simulink model "ComponentSS"  (Simulink 7.5)
settings: Solver=ode45  StartTime=0.0  StopTime=inf  MaxStep=2e-2  RelTol=1e-3
InitFcn:
  | k1=1.5;
  | k2=.4;
  | c1=.5;
  | c2=.001;
  | m1=.1;
  | m2=.002;
  | 
  | A=[0,0,1,0;0,0,0,1;-(k1+k2)/m1,k2/m1,-(c1+c2)/m1,c2/m1;k2/m2,-k2/m2,c2/m2,-c2/m2];
  | B=[0,0;0,0;1/m1,0;0,1/m2];
  | C=eye(4);
  | D=zeros(4,2);
settings Model: Creator=cfadnavi  LastModifiedBy=dmanegol

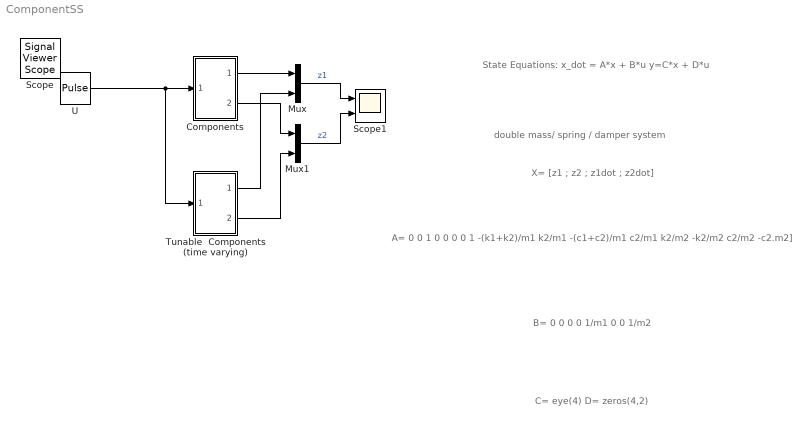
== system ComponentSS ==
  note: State Equations:
      | x_dot = A*x + B*u
      | y=C*x + D*u
  note: X=
      | [z1 ; z2 ; z1dot ; z2dot]
  note: A=
      | 0                  0                   1                 0
      | 0                  0                   0                 1
      | -(k1+k2)/m1     k2/m1   -(c1+c2)/m1    c2/m1
      | k2/m2         -k2/m2         c2/m2         -c2.m2]
  note: B=
      | 0              0
      | 0              0
      | 1/m1        0
      | 0      1/m2
  note: C= eye(4)
      |
      | D= zeros(4,2)
  note: double mass/ spring / damper system
  Components : Subsystem
  Mux : Mux  Inputs=2
  Mux1 : Mux  Inputs=2
  Scope1 : Scope  NumInputPorts=2
      settings: TimeRange=10  YMin=-0.5~-2  YMax=2.5~10
  Tunable  Components (time varying) : Subsystem
  U : DiscretePulseGenerator  PulseType=Time based  Amplitude=[1,1]  Period=[10,10]  PulseWidth=50  PhaseDelay=0  SampleTime=1
  Scope : SignalViewerScope  IOType=viewer  RefreshTime=0.035000
  wires:
  U/1 -> Components/1(In1), Tunable  Components (time varying)/1(In1)
  Components/1(Out1) -> Mux/1
  Mux/1 -> Scope1/1  "z1"
  Mux1/1 -> Scope1/2  "z2"
  Tunable  Components (time varying)/1(Out2) -> Mux/2
  Components/2(Out2) -> Mux1/1
  Tunable  Components (time varying)/2(Out3) -> Mux1/2

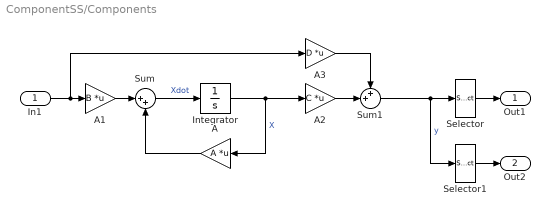
== system ComponentSS/Components ==
  In1 : Inport
  A : Gain  Gain=A  Multiplication=Matrix(K*u)  ParameterDataType=fixdt(1, 16)  ParameterScaling=2^0  OutDataType=fixdt(1, 16)  OutScaling=2^0
  A1 : Gain  Gain=B  Multiplication=Matrix(K*u)  ParameterDataType=fixdt(1, 16)  ParameterScaling=2^0  OutDataType=fixdt(1, 16)  OutScaling=2^0
  A2 : Gain  Gain=C  Multiplication=Matrix(K*u)  ParameterDataType=fixdt(1, 16)  ParameterScaling=2^0  OutDataType=fixdt(1, 16)  OutScaling=2^0
  A3 : Gain  Gain=D  Multiplication=Matrix(K*u)  ParameterDataType=fixdt(1, 16)  ParameterScaling=2^0  OutDataType=fixdt(1, 16)  OutScaling=2^0
  Integrator : Integrator
  Selector : Selector  InputPortWidth=4  IndexOptions=Index vector (dialog)  Indices=1  OutputSizes=1
  Selector1 : Selector  InputPortWidth=4  IndexOptions=Index vector (dialog)  Indices=2  OutputSizes=1
  Sum : Sum  Inputs=|++  OutDataType=fixdt(1, 16)  OutScaling=2^0
  Sum1 : Sum  Inputs=++|  OutDataType=fixdt(1, 16)  OutScaling=2^0
  Out1 : Outport
  Out2 : Outport  Port=2
  wires:
  A/1 -> Sum/2
  Integrator/1 -> A/1, A2/1  "X"
  Sum/1 -> Integrator/1  "Xdot"
  A1/1 -> Sum/1
  A2/1 -> Sum1/2
  A3/1 -> Sum1/1
  In1/1 -> A3/1, A1/1
  Sum1/1 -> Selector/1, Selector1/1  "y"
  Selector/1 -> Out1/1
  Selector1/1 -> Out2/1

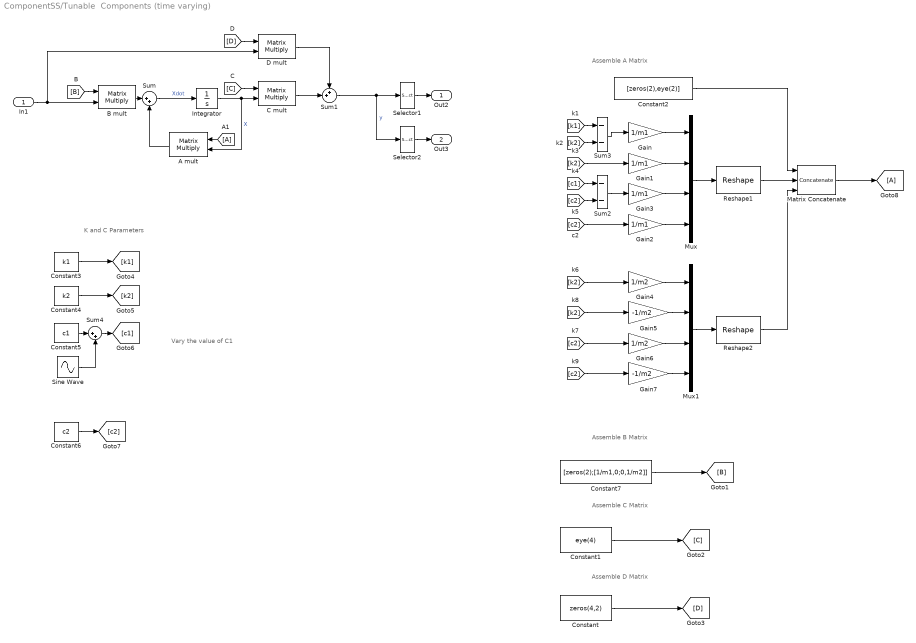
== system ComponentSS/Tunable  Components (time varying) ==
  note: Assemble A Matrix
  note: Assemble B Matrix
  note: Assemble D Matrix
  note: Assemble C Matrix
  note: K and C Parameters
  note: Vary the value of C1
  In1 : Inport
  A mult : Product  Multiplication=Matrix(*)  OutDataType=fixdt(1, 16)  OutScaling=2^0  RndMeth=Zero
  B mult : Product  Multiplication=Matrix(*)  OutDataType=fixdt(1, 16)  OutScaling=2^0  RndMeth=Zero
  C mult : Product  Multiplication=Matrix(*)  OutDataType=fixdt(1, 16)  OutScaling=2^0  RndMeth=Zero
  Constant : Constant  Value=zeros(4,2)  OutDataType=fixdt(1, 16)  OutScaling=2^0
  Constant1 : Constant  Value=eye(4)  OutDataType=fixdt(1, 16)  OutScaling=2^0
  Constant2 : Constant  Value=[zeros(2),eye(2)]  OutDataType=fixdt(1, 16)  OutScaling=2^0
  Constant3 : Constant  Value=k1  OutDataType=fixdt(1, 16)  OutScaling=2^0
  Constant4 : Constant  Value=k2  OutDataType=fixdt(1, 16)  OutScaling=2^0
  Constant5 : Constant  Value=c1  OutDataType=fixdt(1, 16)  OutScaling=2^0
  Constant6 : Constant  Value=c2  OutDataType=fixdt(1, 16)  OutScaling=2^0
  Constant7 : Constant  Value=[zeros(2);[1/m1,0;0,1/m2]]  OutDataType=fixdt(1, 16)  OutScaling=2^0
  D mult : Product  Multiplication=Matrix(*)  OutDataType=fixdt(1, 16)  OutScaling=2^0  RndMeth=Zero
  Gain{,1..3} (4 alike) : Gain  Gain=1/m1  ParameterDataType=fixdt(1, 16)  ParameterScaling=2^0  OutDataType=fixdt(1, 16)  OutScaling=2^0
  Gain4 : Gain  Gain=1/m2  ParameterDataType=fixdt(1, 16)  ParameterScaling=2^0  OutDataType=fixdt(1, 16)  OutScaling=2^0
  Gain5 : Gain  Gain=-1/m2  ParameterDataType=fixdt(1, 16)  ParameterScaling=2^0  OutDataType=fixdt(1, 16)  OutScaling=2^0
  Gain6 : Gain  Gain=1/m2  ParameterDataType=fixdt(1, 16)  ParameterScaling=2^0  OutDataType=fixdt(1, 16)  OutScaling=2^0
  Gain7 : Gain  Gain=-1/m2  ParameterDataType=fixdt(1, 16)  ParameterScaling=2^0  OutDataType=fixdt(1, 16)  OutScaling=2^0
  Integrator : Integrator
  Matrix Concatenate : Concatenate  NumInputs=3  Mode=Multidimensional array
  Mux : Mux
  Mux1 : Mux
  Reshape1 : Reshape  OutputDimensionality=Row vector (2-D)  OutputDimensions=[2, 2]
  Reshape2 : Reshape  OutputDimensionality=Row vector (2-D)  OutputDimensions=[2, 2]
  Selector1 : Selector  InputPortWidth=4  IndexOptions=Index vector (dialog)  Indices=1  OutputSizes=1
  Selector2 : Selector  InputPortWidth=4  IndexOptions=Index vector (dialog)  Indices=2  OutputSizes=1
  Sine Wave : Sin  Amplitude=.4  Bias=0  Frequency=2e-2  Phase=0  Samples=10  SampleTime=0  Offset=0
  Sum : Sum  Inputs=|++  OutDataType=fixdt(1, 16)  OutScaling=2^0
  Sum1 : Sum  Inputs=++|  OutDataType=fixdt(1, 16)  OutScaling=2^0
  Sum2 : Sum  Inputs=--  OutDataType=fixdt(1, 16)  OutScaling=2^0
  Sum3 : Sum  Inputs=--  OutDataType=fixdt(1, 16)  OutScaling=2^0
  Sum4 : Sum  Inputs=|++  OutDataType=fixdt(1, 16)  OutScaling=2^0
  Out2 : Outport
  Out3 : Outport  Port=2
  wires:
  Sum1/1 -> Selector2/1, Selector1/1  "y"
  In1/1 -> B mult/2, D mult/2
  D mult/1 -> Sum1/1
  C mult/1 -> Sum1/2
  B mult/1 -> Sum/1
  Sum/1 -> Integrator/1  "Xdot"
  Integrator/1 -> A mult/2, C mult/2  "X"
  A mult/1 -> Sum/2
  [B] -> B mult/1
  [A] -> A mult/1
  [C] -> C mult/1
  [D] -> D mult/1
  Constant/1 -> [D]
  Constant1/1 -> [C]
  [k1] -> Sum3/1
  [k2] -> Sum3/2
  Constant3/1 -> [k1]
  Constant4/1 -> [k2]
  Constant6/1 -> [c2]
  Sum3/1 -> Gain/1
  Gain/1 -> Mux/1
  [k2] -> Gain1/1
  Gain1/1 -> Mux/2
  [c2] -> Gain2/1
  [c1] -> Sum2/1
  Sum2/1 -> Gain3/1
  Gain3/1 -> Mux/3
  [c2] -> Sum2/2
  Gain2/1 -> Mux/4
  Gain4/1 -> Mux1/1
  [k2] -> Gain5/1
  Gain5/1 -> Mux1/2
  Gain6/1 -> Mux1/3
  Gain7/1 -> Mux1/4
  [k2] -> Gain4/1
  [c2] -> Gain7/1
  [c2] -> Gain6/1
  Mux/1 -> Reshape1/1
  Mux1/1 -> Reshape2/1
  Constant2/1 -> Matrix Concatenate/1
  Reshape1/1 -> Matrix Concatenate/2
  Reshape2/1 -> Matrix Concatenate/3
  Matrix Concatenate/1 -> [A]
  Selector1/1 -> Out2/1
  Selector2/1 -> Out3/1
  Constant7/1 -> [B]
  Constant5/1 -> Sum4/1
  Sum4/1 -> [c1]
  Sine Wave/1 -> Sum4/2
